simulink model "fuzzy_faja"  (R2021a)
settings: Solver=VariableStepAuto  StartTime=0.0  StopTime=20  FixedStep=0.001  RelTol=1e-3
libraries: fuzblock x1
settings Model: Creator=Bremdows  LastModifiedBy=Bremdows

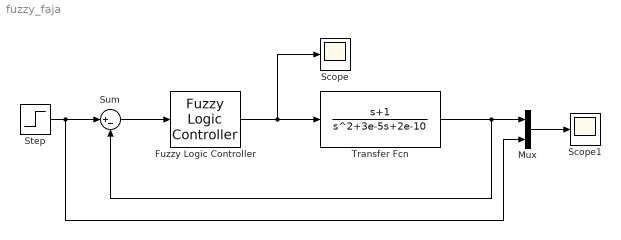
== system fuzzy_faja ==
  Fuzzy Logic Controller : fuzblock/Fuzzy Logic  Controller  FIS='fuzzy_faja_mandani.fis'  OutputSampleNumber=101  DataType=double  FuzzifiedInputs=off  RuleFiringStrengths=off  RuleOutputs=off  AggregatedOutputs=off  SimulateUsing=Interpreted execution  OutOfRangeInputValueMessage=warning  NoRuleFiredMessage=warning  EmptyOutputFuzzySetMessage=warning
  Mux : Mux  Inputs=2
  Scope : Scope
  Scope1 : Scope
  Step : Step  Time=0  After=0.1  SampleTime=0
  Sum : Sum  Inputs=|+-
  Transfer Fcn : TransferFcn  Numerator=[1 1]  Denominator=[1 3e-5 2e-10]
  wires:
  Transfer Fcn/1 -> Sum/2, Mux/1
  Mux/1 -> Scope1/1
  Fuzzy Logic Controller/1 -> Scope/1, Transfer Fcn/1
  Sum/1 -> Fuzzy Logic Controller/1
  Step/1 -> Mux/2, Sum/1
